simulink model "counters_amol_sir"  (R2020a)
settings: Solver=VariableStepAuto  StartTime=0.0  StopTime=100  RelTol=1e-3
libraries: simulink x17
settings Model: SnapshotBufferSize=1  SnapshotInterval=1  Creator=Pratik shinde  LastModifiedBy=rushikesh bharti
settings OptimizationCC: DefaultParameterBehavior=Inlined  EnhancedBackFolding=on  PassReuseOutputArgsAs=Individual arguments  ZeroExternalMemoryAtStartup=off  ZeroInternalMemoryAtStartup=off  OptimizeBlockOrder=speed  DifferentSizesBufferReuse=on  OptimizationCustomize=off  EfficientTunableParamExpr=on
settings DebuggingCC: ParameterTunabilityLossMsg=error
settings SFSimCC: MATLABDynamicMemAlloc=off
settings RTWCC: SystemTargetFile=ert.tlc  TemplateMakefile=ert_default_tmf
settings CodeAppCC: ForceParamTrailComments=on  IgnoreCustomStorageClasses=off  OperatorAnnotations=on  SimulinkDataObjDesc=on  SFDataObjDesc=on  InsertBlockDesc=on
settings ERTTargetCC: TargetLangStandard=C99 (ISO)  GenerateSampleERTMain=on  InlinedParameterPlacement=NonHierarchical  ERTCustomFileTemplate=example_file_process.tlc

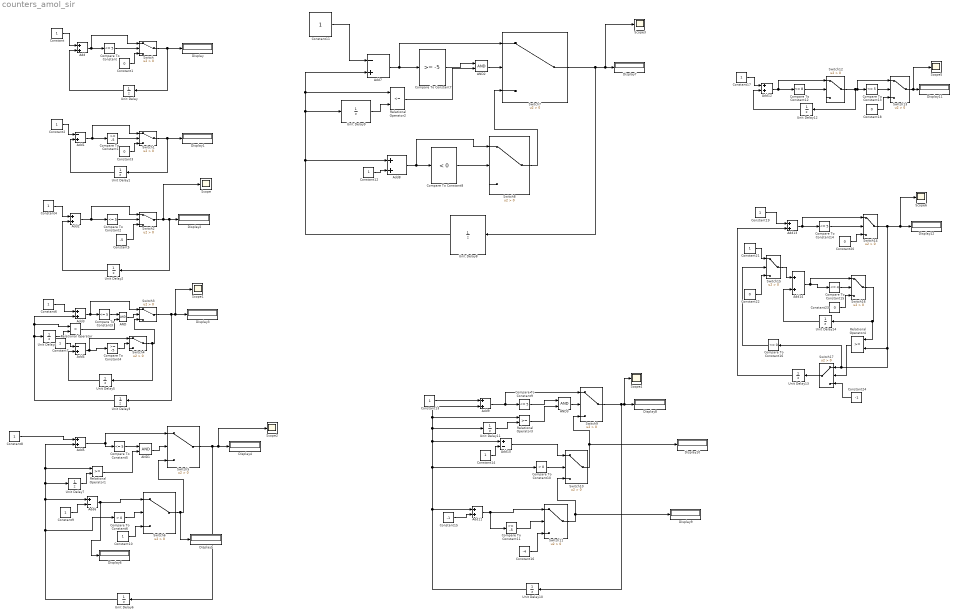
== system counters_amol_sir ==
  AND{,1..3} (4 alike) : Logic  AllPortsSameDT=off  OutDataTypeStr=boolean
  Add{,2..3,5,8..9,11..14} (10 alike) : Sum
  Add1 : Sum  Inputs=-+
  Add10 : Sum  Inputs=+-
  Add4 : Sum  Inputs=-+
  Add6 : Sum  Inputs=+-
  Add7 : Sum  Inputs=-+
  Compare To Constant{,2..3,5,9,13..14} (7 alike) : simulink/Logic and Bit Operations/Compare To Constant  relop=<=  const=5  OutDataTypeStr=boolean
  Compare To Constant{1,4,7,11} (4 alike) : simulink/Logic and Bit Operations/Compare To Constant  relop=>=  const=-5  OutDataTypeStr=boolean
  Compare To Constant10 : simulink/Logic and Bit Operations/Compare To Constant  relop=>  const=0  OutDataTypeStr=boolean
  Compare To Constant12 : simulink/Logic and Bit Operations/Compare To Constant  relop=<=  const=8  OutDataTypeStr=boolean
  Compare To Constant15 : simulink/Logic and Bit Operations/Compare To Constant  relop=<=  const=4  OutDataTypeStr=boolean
  Compare To Constant16 : simulink/Logic and Bit Operations/Compare To Constant  relop=<=  const=0  OutDataTypeStr=boolean
  Compare To Constant6 : simulink/Logic and Bit Operations/Compare To Constant  relop=>  const=0  OutDataTypeStr=boolean
  Compare To Constant8 : simulink/Logic and Bit Operations/Compare To Constant  relop=<  const=0  OutDataTypeStr=boolean
  Constant{,2,4,6..14,17,19,21} (15 alike) : Constant
  Constant{1,3,18,20,22..23} (6 alike) : Constant  Value=0
  Constant15 : Constant  Value=-1
  Constant16 : Constant  Value=-4
  Constant24 : Constant  Value=-1
  Constant5 : Constant  Value=-5
  Display{,1..12} (13 alike) : Display
  Relational Operator : RelationalOperator  Operator=>  OutDataTypeStr=boolean  RndMeth=Simplest
  Relational Operator1 : RelationalOperator  OutDataTypeStr=boolean  RndMeth=Simplest
  Relational Operator2 : RelationalOperator  Operator=<=  OutDataTypeStr=boolean  RndMeth=Simplest
  Relational Operator3 : RelationalOperator  OutDataTypeStr=boolean  RndMeth=Simplest
  Relational Operator4 : RelationalOperator  OutDataTypeStr=boolean  RndMeth=Simplest
  Scope{,1..6} (7 alike) : Scope
  Switch{,1..17} (18 alike) : Switch  Criteria=u2 > Threshold
  Unit Delay{,2..3,6..7,10..14} (10 alike) : UnitDelay  InitialCondition=-1  SampleTime=-1  HasFrameUpgradeWarning=on
  Unit Delay{1,5,8..9} (4 alike) : UnitDelay  InitialCondition=1  SampleTime=-1  HasFrameUpgradeWarning=on
  Unit Delay4 : UnitDelay  InitialCondition=-2  SampleTime=-1  HasFrameUpgradeWarning=on
  wires:
  Constant/1 -> Add/1
  Add/1 -> Switch/1, Compare To Constant/1
  Compare To Constant/1 -> Switch/2
  Switch/1 -> Display/1, Unit Delay/1
  Unit Delay/1 -> Add/2
  Constant1/1 -> Switch/3
  Add1/1 -> Switch1/1, Compare To Constant1/1
  Compare To Constant1/1 -> Switch1/2
  Switch1/1 -> Unit Delay1/1, Display1/1
  Unit Delay1/1 -> Add1/2
  Constant2/1 -> Add1/1
  Constant3/1 -> Switch1/3
  Constant4/1 -> Add2/1
  Add2/1 -> Switch2/1, Compare To Constant2/1
  Compare To Constant2/1 -> Switch2/2
  Switch2/1 -> Scope/1, Unit Delay2/1, Display2/1
  Unit Delay2/1 -> Add2/2
  Constant5/1 -> Switch2/3
  Constant6/1 -> Add3/1
  Add3/1 -> Switch3/1, Compare To Constant3/1
  Switch3/1 -> Unit Delay3/1, Scope1/1, Display3/1
  Unit Delay3/1 -> Unit Delay4/1, Relational Operator/1, Add3/2
  Switch4/1 -> Unit Delay5/1, Switch3/3
  Constant7/1 -> Add4/1
  Add4/1 -> Switch4/1, Compare To Constant4/1
  Compare To Constant4/1 -> Switch4/2
  Compare To Constant3/1 -> AND/1
  AND/1 -> Switch3/2
  Relational Operator/1 -> AND/2
  Unit Delay4/1 -> Relational Operator/2
  Unit Delay5/1 -> Add4/2
  Switch5/1 -> Unit Delay6/1, Scope2/1, Display4/1
  Add5/1 -> Compare To Constant5/1, Switch5/1
  Constant8/1 -> Add5/1
  Unit Delay6/1 -> Compare To Constant6/1, Relational Operator1/1, Add5/2, Unit Delay7/1, Add6/1
  Constant9/1 -> Add6/2
  Switch6/1 -> Display5/1, Switch5/3
  Compare To Constant5/1 -> AND1/1
  AND1/1 -> Switch5/2
  Relational Operator1/1 -> AND1/2
  Unit Delay7/1 -> Relational Operator1/2
  Add6/1 -> Display6/1, Switch6/1
  Compare To Constant6/1 -> Switch6/2
  Constant10/1 -> Switch6/3
  Switch7/1 -> Unit Delay8/1, Scope3/1, Display7/1
  Add7/1 -> Switch7/1, Compare To Constant7/1
  Constant11/1 -> Add7/1
  Unit Delay8/1 -> Add7/2, Relational Operator2/1, Unit Delay9/1, Add8/1
  Unit Delay9/1 -> Relational Operator2/2
  Constant12/1 -> Add8/2
  Add8/1 -> Switch8/1, Compare To Constant8/1
  Compare To Constant8/1 -> Switch8/2
  Switch8/1 -> Switch7/3
  Compare To Constant7/1 -> AND2/1
  Relational Operator2/1 -> AND2/2
  AND2/1 -> Switch7/2
  Constant13/1 -> Add9/1
  Add9/1 -> Switch9/1, Compare To Constant9/1
  Switch9/1 -> Unit Delay10/1, Scope4/1, Display8/1
  Unit Delay10/1 -> Compare To Constant10/1, Add10/1, Unit Delay11/1, Relational Operator3/1, Add9/2, Add11/1
  Compare To Constant10/1 -> Switch10/2
  Constant14/1 -> Add10/2
  Add10/1 -> Switch10/1
  Switch10/1 -> Switch9/3, Display10/1
  Compare To Constant9/1 -> AND3/1
  Unit Delay11/1 -> Relational Operator3/2
  Relational Operator3/1 -> AND3/2
  AND3/1 -> Switch9/2
  Switch11/1 -> Switch10/3, Display9/1
  Constant15/1 -> Add11/2
  Compare To Constant11/1 -> Switch11/2
  Add11/1 -> Compare To Constant11/1, Switch11/1
  Constant16/1 -> Switch11/3
  Add12/1 -> Switch12/1, Compare To Constant12/1
  Compare To Constant12/1 -> Switch12/2
  Constant17/1 -> Add12/1
  Unit Delay12/1 -> Add12/2
  Switch12/1 -> Unit Delay12/1, Switch13/1, Compare To Constant13/1
  Compare To Constant13/1 -> Switch13/2
  Constant18/1 -> Switch13/3
  Switch13/1 -> Scope5/1, Display11/1
  Add13/1 -> Switch14/1, Compare To Constant14/1
  Constant19/1 -> Add13/1
  Compare To Constant14/1 -> Switch14/2
  Switch14/1 -> Scope6/1, Display12/1, Compare To Constant16/1, Switch17/1, Relational Operator4/2
  Unit Delay13/1 -> Add13/2
  Constant20/1 -> Switch14/3
  Constant22/1 -> Switch15/3
  Constant21/1 -> Switch15/1
  Switch15/1 -> Add14/1
  Compare To Constant15/1 -> Switch16/2
  Add14/1 -> Switch16/1, Compare To Constant15/1
  Constant23/1 -> Switch16/3
  Switch16/1 -> Relational Operator4/1, Unit Delay14/1
  Unit Delay14/1 -> Add14/2
  Relational Operator4/1 -> Switch17/2
  Constant24/1 -> Switch17/3
  Switch17/1 -> Unit Delay13/1
  Compare To Constant16/1 -> Switch15/2
